simulink model "stateMachineAndGaitPlayback"  (R2016b)
settings: Solver=FixedStepAuto  StartTime=0.0  StopTime=10  FixedStep=0.002  RelTol=1e-3
undefined symbols (not defined in the file or in its folder): Leg, StepType
libraries: VariousLibrary x2, GaitHandler x1, StatemachineMARCH x1
settings Model: DataDictionary=ModelDictionary.sldd  Creator=Taeke  LastModifiedBy=Taeke

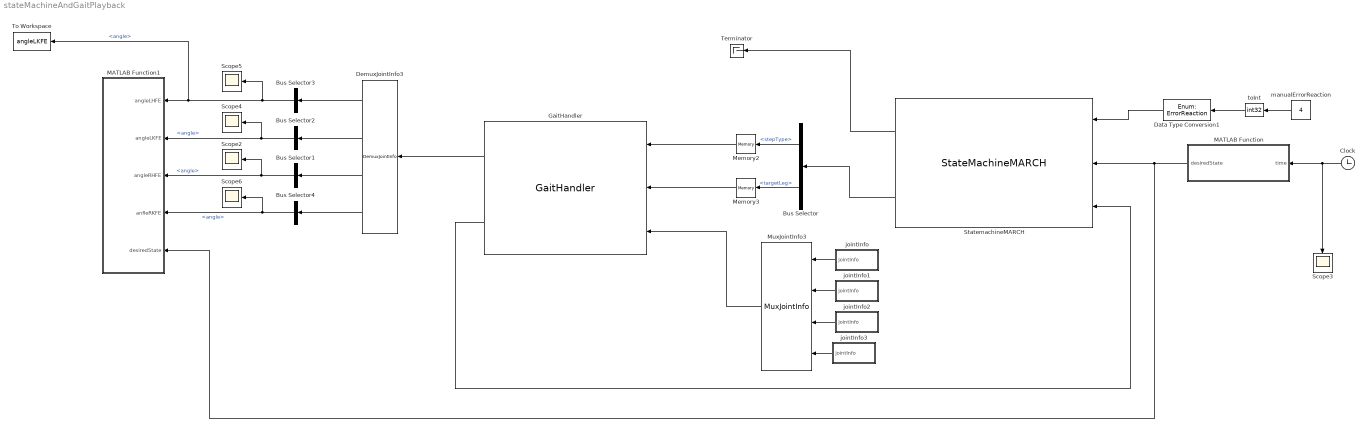
== system stateMachineAndGaitPlayback ==
  Bus Selector : BusSelector  OutputSignals=stepType,targetLeg
  Bus Selector{1..4} (4 alike) : BusSelector  OutputSignals=angle
  Clock : Clock
  Data Type Conversion1 : DataTypeConversion  OutDataTypeStr=Enum: ErrorReaction
  DemuxJointInfo3 : VariousLibrary/DemuxJointInfo
  GaitHandler : GaitHandler/GaitHandler
  MATLAB Function : MATLAB Function  TreatAsAtomicUnit=on
  MATLAB Function1 : MATLAB Function  TreatAsAtomicUnit=on
  Memory2 : Memory  X0=StepType.NOSTEP
  Memory3 : Memory  X0=Leg.NONE
  MuxJointInfo3 : VariousLibrary/MuxJointInfo
  Scope{2..6} (5 alike) : Scope
  StatemachineMARCH : StatemachineMARCH/StateMachineMARCH
  Terminator : Terminator
  To Workspace : ToWorkspace  VariableName=angleLKFE  SaveFormat=Timeseries  SampleTime=-1
  jointInfo : Subsystem
  jointInfo1 : Subsystem
  jointInfo2 : Subsystem
  jointInfo3 : Subsystem
  manualErrorReaction : Constant  Value=4
  toInt : DataTypeConversion  OutDataTypeStr=int32
  wires:
  StatemachineMARCH/2 -> Bus Selector/1
  Bus Selector/1 -> Memory2/1  "<stepType>"
  Bus Selector/2 -> Memory3/1  "<targetLeg>"
  Memory2/1 -> GaitHandler/1
  Memory3/1 -> GaitHandler/2
  StatemachineMARCH/1 -> Terminator/1
  manualErrorReaction/1 -> toInt/1
  toInt/1 -> Data Type Conversion1/1
  Data Type Conversion1/1 -> StatemachineMARCH/1
  GaitHandler/2 -> StatemachineMARCH/3
  Clock/1 -> Scope3/1, MATLAB Function/1(time)
  MATLAB Function/1(desiredState) -> StatemachineMARCH/2, MATLAB Function1/5(desiredState)
  MuxJointInfo3/1 -> GaitHandler/3
  Bus Selector1/1 -> Scope2/1, MATLAB Function1/3(angleRHFE)  "<angle>"
  DemuxJointInfo3/3 -> Bus Selector1/1
  GaitHandler/1 -> DemuxJointInfo3/1
  Bus Selector2/1 -> MATLAB Function1/2(angleLKFE), Scope4/1  "<angle>"
  DemuxJointInfo3/2 -> Bus Selector2/1
  Bus Selector3/1 -> To Workspace/1, MATLAB Function1/1(angleLHFE), Scope5/1  "<angle>"
  DemuxJointInfo3/1 -> Bus Selector3/1
  Bus Selector4/1 -> Scope6/1, MATLAB Function1/4(anfleRKFE)  "<angle>"
  DemuxJointInfo3/4 -> Bus Selector4/1
  jointInfo/1(jointInfo) -> MuxJointInfo3/1
  jointInfo1/1(jointInfo) -> MuxJointInfo3/2
  jointInfo2/1(jointInfo) -> MuxJointInfo3/3
  jointInfo3/1(jointInfo) -> MuxJointInfo3/4

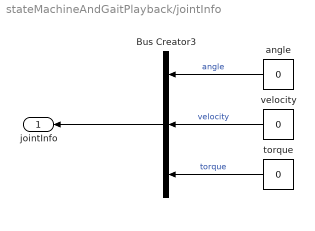
== system stateMachineAndGaitPlayback/jointInfo ==
  Bus Creator3 : BusCreator  Inputs=3  OutDataTypeStr=Bus: JointDynamics  NonVirtualBus=on
  angle : Constant  Value=0
  torque : Constant  Value=0
  velocity : Constant  Value=0
  jointInfo : Outport
  wires:
  Bus Creator3/1 -> jointInfo/1
  angle/1 -> Bus Creator3/1  "angle"
  velocity/1 -> Bus Creator3/2  "velocity"
  torque/1 -> Bus Creator3/3  "torque"

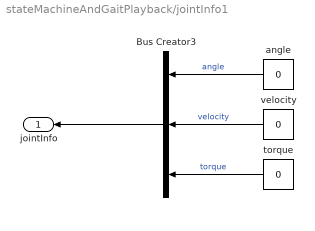
== system stateMachineAndGaitPlayback/jointInfo1 ==
  Bus Creator3 : BusCreator  Inputs=3  OutDataTypeStr=Bus: JointDynamics  NonVirtualBus=on
  angle : Constant  Value=0
  torque : Constant  Value=0
  velocity : Constant  Value=0
  jointInfo : Outport
  wires:
  Bus Creator3/1 -> jointInfo/1
  angle/1 -> Bus Creator3/1  "angle"
  velocity/1 -> Bus Creator3/2  "velocity"
  torque/1 -> Bus Creator3/3  "torque"

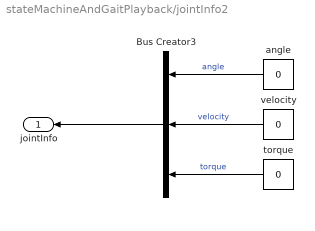
== system stateMachineAndGaitPlayback/jointInfo2 ==
  Bus Creator3 : BusCreator  Inputs=3  OutDataTypeStr=Bus: JointDynamics  NonVirtualBus=on
  angle : Constant  Value=0
  torque : Constant  Value=0
  velocity : Constant  Value=0
  jointInfo : Outport
  wires:
  Bus Creator3/1 -> jointInfo/1
  angle/1 -> Bus Creator3/1  "angle"
  velocity/1 -> Bus Creator3/2  "velocity"
  torque/1 -> Bus Creator3/3  "torque"

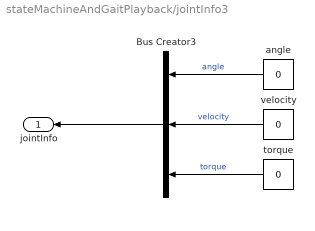
== system stateMachineAndGaitPlayback/jointInfo3 ==
  Bus Creator3 : BusCreator  Inputs=3  OutDataTypeStr=Bus: JointDynamics  NonVirtualBus=on
  angle : Constant  Value=0
  torque : Constant  Value=0
  velocity : Constant  Value=0
  jointInfo : Outport
  wires:
  Bus Creator3/1 -> jointInfo/1
  angle/1 -> Bus Creator3/1  "angle"
  velocity/1 -> Bus Creator3/2  "velocity"
  torque/1 -> Bus Creator3/3  "torque"

== matlab function stateMachineAndGaitPlayback/MATLAB Function1 ==
  data: angleLHFE input; angleLKFE input; angleRHFE input; anfleRKFE input; desiredState input
function fcn(angleLHFE, angleLKFE, angleRHFE, anfleRKFE, desiredState)
%figure
%plot(angleLHFE)

== matlab function stateMachineAndGaitPlayback/MATLAB Function ==
  data: time input; desiredState output
function desiredState = fcn(time)
desiredState = drunkUser(time);
